simulink model "testEmojis"  (R2024a)
settings: Solver=FixedStepAuto  StartTime=0  StopTime=10.0  RelTol=1e-3
PreLoadFcn:
  | %Not good 👍
settings Model: Creator=grouleau  LastModifiedBy=grouleau
settings OptimizationCC: DefaultParameterBehavior=Inlined  EnhancedBackFolding=on  PassReuseOutputArgsAs=Individual arguments  ZeroExternalMemoryAtStartup=off  ZeroInternalMemoryAtStartup=off  OptimizeBlockOrder=speed  DifferentSizesBufferReuse=on  OptimizationCustomize=off  EfficientTunableParamExpr=on
settings DebuggingCC: ParameterTunabilityLossMsg=error
settings SFSimCC: MATLABDynamicMemAlloc=off
settings RTWCC: Description=Embedded Coder  SystemTargetFile=ert.tlc  TemplateMakefile=ert_default_tmf
settings CodeAppCC: ForceParamTrailComments=on  IgnoreCustomStorageClasses=off  OperatorAnnotations=on  SimulinkDataObjDesc=on  SFDataObjDesc=on  InsertBlockDesc=on
settings ERTTargetCC: TargetLangStandard=C99 (ISO)  GenerateSampleERTMain=on  InlinedParameterPlacement=NonHierarchical  ERTCustomFileTemplate=example_file_process.tlc

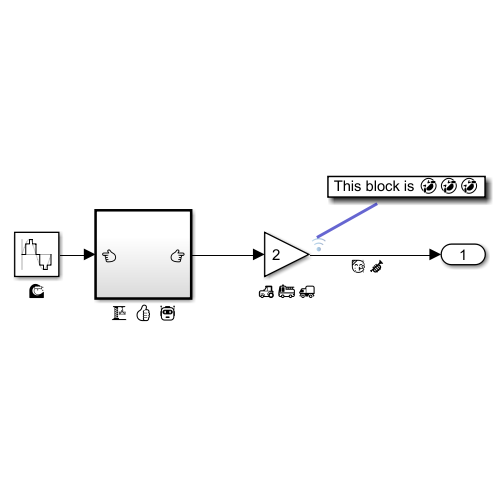
[thumbnail: Simulink's stored preview of the top-level diagram]
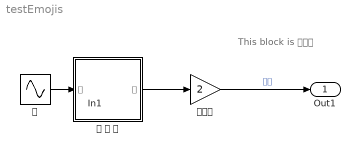
== system testEmojis ==
  note: This block is 🤣🤣🤣
  In1 : Inport
  🌊 : Sin  SampleTime=0.01
  🏗️ 👍 🤖 : Subsystem  TreatAsAtomicUnit=on
      settings: RTWFcnNameOpts=Use subsystem name  RTWFileNameOpts=Use subsystem name
  🚜🚒🚚 : Gain  Gain=2
  Out1 : Outport
  wires:
  🚜🚒🚚/1 -> Out1/1  "🥳🎺"
  🏗️ 👍 🤖/1(👉) -> 🚜🚒🚚/1
  🌊/1 -> 🏗️ 👍 🤖/1(👈)

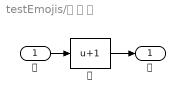
== system testEmojis/🏗️ 👍 🤖 ==
  👈 : Inport
  🏗️ : Bias  Bias=1  SaturateOnIntegerOverflow=off
  👉 : Outport
  wires:
  👈/1 -> 🏗️/1
  🏗️/1 -> 👉/1
